simulink model "MPC_no_constraints_sim"  (R2022a)
settings: Solver=VariableStepAuto  StartTime=0.0  StopTime=Ts  RelTol=1e-3
values from neighbouring files (symbols this model uses):
  C_states = eye(length(A))    [main.m]    (also in main_cessna.m = eye(4))
  D_states = zeros(length(B), 1)    [main.m]
  P_MPC = Q_LQ_d    [main.m]
  Q_MPC = Q_LQ_d    [main.m]
  R_MPC = R_LQ_d    (= 10000)    [main.m]
  SetN = [20 30 90]    [main.m]
  sysd = c2d(sys,T_sampling)    [main.m]
  T_sampling = 2*pi/omega_sampling    [main.m]
  x0 = [deg2rad(0) deg2rad(15) 0 -300]    [main.m]    (also in main_cessna.m = [0 0 0 5000])
  x_ref = [0 0 0 0]    [main.m]
undefined symbols (not defined in the file or in its folder): k_LQ_d, MPC_no_constraints
settings Model: Creator=g_mor  LastModifiedBy=g_mor

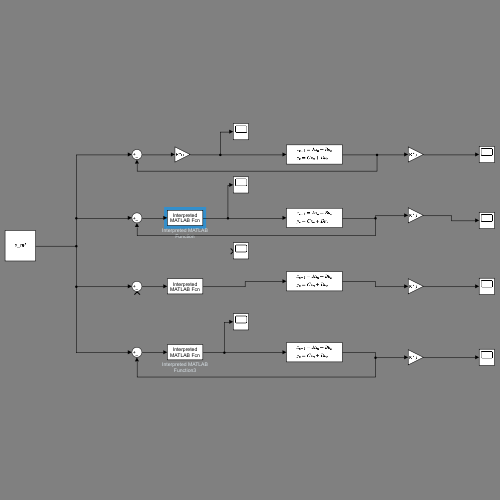
[thumbnail: Simulink's stored preview of the top-level diagram]
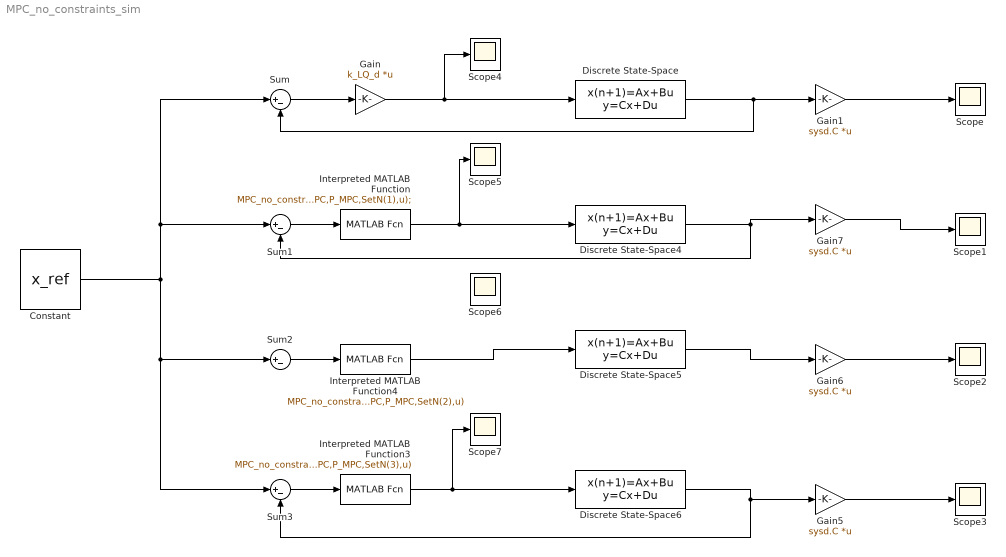
== system MPC_no_constraints_sim ==
  Constant : Constant  Value=x_ref
  Discrete State-Space{,4..6} (4 alike) : DiscreteStateSpace  A=sysd.A  B=sysd.B  C=C_states  D=D_states  InitialCondition=x0  SampleTime=T_sampling
  Gain : Gain  Gain=k_LQ_d  Multiplication=Matrix(K*u)
  Gain{1,5..7} (4 alike) : Gain  Gain=sysd.C  Multiplication=Matrix(K*u)
  Interpreted MATLAB Function : MATLABFcn  MATLABFcn=MPC_no_constraints(sysd.A,sysd.B,Q_MPC,R_MPC,P_MPC,SetN(1),u);  OutputDimensions=1
  Interpreted MATLAB Function3 : MATLABFcn  MATLABFcn=MPC_no_constraints(sysd.A,sysd.B,Q_MPC,R_MPC,P_MPC,SetN(3),u)  OutputDimensions=1
  Interpreted MATLAB Function4 : MATLABFcn  MATLABFcn=MPC_no_constraints(sysd.A,sysd.B,Q_MPC,R_MPC,P_MPC,SetN(2),u)  OutputDimensions=1
  Scope{,1..7} (8 alike) : Scope
  Sum{,1..3} (4 alike) : Sum  Inputs=|+-
  wires:
  Sum/1 -> Gain/1
  Gain/1 -> Scope4/1, Discrete State-Space/1
  Discrete State-Space/1 -> Sum/2, Gain1/1
  Gain1/1 -> Scope/1
  Sum1/1 -> Interpreted MATLAB Function/1
  Interpreted MATLAB Function/1 -> Discrete State-Space4/1, Scope5/1
  Discrete State-Space4/1 -> Gain7/1, Sum1/2
  Gain7/1 -> Scope1/1
  Sum2/1 -> Interpreted MATLAB Function4/1
  Interpreted MATLAB Function4/1 -> Discrete State-Space5/1
  Discrete State-Space5/1 -> Gain6/1
  Gain6/1 -> Scope2/1
  Sum3/1 -> Interpreted MATLAB Function3/1
  Interpreted MATLAB Function3/1 -> Discrete State-Space6/1, Scope7/1
  Discrete State-Space6/1 -> Gain5/1, Sum3/2
  Gain5/1 -> Scope3/1
  Constant/1 -> Sum3/1, Sum2/1, Sum1/1, Sum/1
